simulink library "QuadModelLib2017b"  (R2017b)
settings: Solver=VariableStepAuto  StartTime=0.0  StopTime=10.0  RelTol=1e-3
values from neighbouring files (symbols this model uses):
  ModelParam_envAltitude = -50    [Init.m]
  ModelParam_noiseGPSSampTime = 0.2    [Init.m]
  ModelParam_noisePowerIMU = 0    [Init.m]
  ModelParam_timeSampBaro = 0.01    [Init.m]
  MotorFault1 = MotorFaultTemp    [Init.m]
undefined symbols (not defined in the file or in its folder): BatteryFault, Earth, F, FaultParamAPI, Light, LoadFault, MIL, ModelParam_noiseLowPassFilterCoeAccel, ModelParam_noiseLowPassFilterCoeGyro, Moderate, PropFault, SensorFault, WGS84, WindFault
libraries: aerolibwind2 x5, simulink x2, aerolibtransform2 x1, aerolibasang x1, aerolibatmos2 x1, aerolibnav x1, aerolibgravity2 x1
(part 2 of 2)

== matlab function QuadModelLib2017b/WindFault/FaultParamsExtract ==
  settings: updateMethod=DISCRETE
  data: FaultID input; inInts input; hasFault_ConstWind output; inFloats input; FaultParam output
function [hasFault_ConstWind, FaultParam] = fcn(FaultID,inInts,inFloats)
persistent hFault;
persistent fParam;

if isempty(hFault)
    hFault=false;
end
if isempty(fParam)
    fParam=zeros(20,1);
end

hFaultTmp=false;
fParamTmp=zeros(20,1);
j=1;
for i=1:8
    if inInts(i) == FaultID
        hFaultTmp=true;
        fParamTmp(2*j-1)=inFloats(2*i-1);
        fParamTmp(2*j)=inFloats(2*i);
        j=j+1;
    end
end
if hFaultTmp
    hFault=hFaultTmp;
    fParamTmp(17:20) = inFloats(17:20);
    fParam=fParamTmp;
end

hasFault_ConstWind=hFault;
FaultParam=fParam;

== matlab function QuadModelLib2017b/WindFault/FaultParamsExtract2 ==
  settings: updateMethod=DISCRETE
  data: FaultID input; inInts input; hasFault_TurbWind output; inFloats input; FaultParam output
function [hasFault_TurbWind, FaultParam] = fcn(FaultID,inInts,inFloats)
persistent hFault;
persistent fParam;

if isempty(hFault)
    hFault=false;
end
if isempty(fParam)
    fParam=zeros(20,1);
end

hFaultTmp=false;
fParamTmp=zeros(20,1);
j=1;
for i=1:8
    if inInts(i) == FaultID
        hFaultTmp=true;
        fParamTmp(2*j-1)=inFloats(2*i-1);
        fParamTmp(2*j)=inFloats(2*i);
        j=j+1;
    end
end
if hFaultTmp
    hFault=hFaultTmp;
    fParamTmp(17:20) = inFloats(17:20);
    fParam=fParamTmp;
end

hasFault_TurbWind=hFault;
FaultParam=fParam;

== matlab function QuadModelLib2017b/WindFault/FaultParamsExtract3 ==
  settings: updateMethod=DISCRETE
  data: FaultID input; inInts input; hasFault_SheerWind output; inFloats input; FaultParam output
function [hasFault_SheerWind, FaultParam] = fcn(FaultID,inInts,inFloats)
persistent hFault;
persistent fParam;

if isempty(hFault)
    hFault=false;
end
if isempty(fParam)
    fParam=zeros(20,1);
end

hFaultTmp=false;
fParamTmp=zeros(20,1);
j=1;
for i=1:8
    if inInts(i) == FaultID
        hFaultTmp=true;
        fParamTmp(2*j-1)=inFloats(2*i-1);
        fParamTmp(2*j)=inFloats(2*i);
        j=j+1;
    end
end
if hFaultTmp
    hFault=hFaultTmp;
    fParamTmp(17:20) = inFloats(17:20);
    fParam=fParamTmp;
end

hasFault_SheerWind=hFault;
FaultParam=fParam;

== matlab function QuadModelLib2017b/SensorFault/baro NoiseFun ==
  data: isbyroFault input; y output; baroFaultParam input
function y = fcn(isbyroFault,baroFaultParam)

y = 0;
if isbyroFault
    y = baroFaultParam(1);
end

== matlab function QuadModelLib2017b/GPSFault/AccNoiseSwitch1/Acc NoiseFun ==
  data: u input; y output; isAccFault input; AccFaultParams input
function y = fcn(u,isAccFault,AccFaultParams)

y = 0.3*u;

if isAccFault
    y = (0.3+0.7*AccFaultParams(1))*u;
end
